simulink model "pantilt_robot"  (R2020a)
settings: Solver=VariableStepAuto  StartTime=0.0  StopTime=10.0  RelTol=1e-3
undefined symbols (not defined in the file): B, J, j, K, Kd, Ki, Kp, La, N, Ra, Ti, Tt
settings Model: Creator=nikkiepedersen  LastModifiedBy=nikkiepedersen

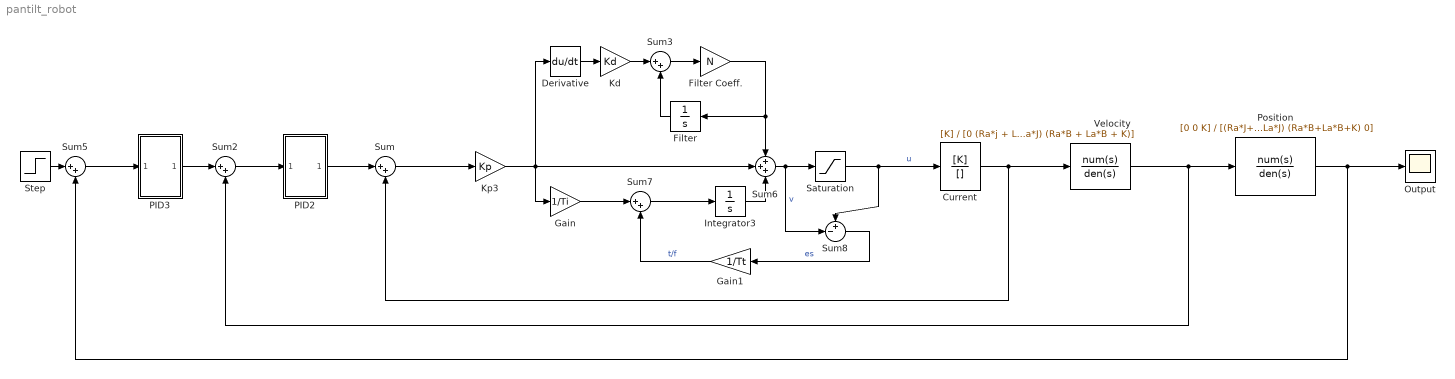
== system pantilt_robot ==
  " Kd" : Gain  Gain=Kd
  Current : TransferFcn  Numerator=[K]  Denominator=[]
  Derivative : Derivative
  Filter : Integrator
  Filter Coeff. : Gain  Gain=N
  Gain : Gain  Gain=1/Ti
  Gain1 : Gain  Gain=1/Tt
  Integrator3 : Integrator
  Kp3 : Gain  Gain=Kp
  Output : Scope
  PID2 : Subsystem
  PID3 : Subsystem
  Position : TransferFcn  Numerator=[0 0 K]  Denominator=[(Ra*J+La*J) (Ra*B+La*B+K) 0]
  Saturation : Saturate
  Step : Step  SampleTime=0
  Sum{,2..3,5,7} (5 alike) : Sum  Inputs=|++
  Sum6 : Sum  Inputs=+++
  Sum8 : Sum  Inputs=+-|
  Velocity : TransferFcn  Numerator=[K]  Denominator=[0 (Ra*j + La*J) (Ra*B + La*B + K)]
  wires:
  Sum/1 -> Kp3/1
  Current/1 -> Velocity/1, Sum/2
  Step/1 -> Sum5/1
  Velocity/1 -> Position/1, Sum2/2
  Position/1 -> Output/1, Sum5/2
  Saturation/1 -> Sum8/1, Current/1  "u"
  Sum7/1 -> Integrator3/1
  Gain/1 -> Sum7/1
  Integrator3/1 -> Sum6/3
  Sum6/1 -> Saturation/1, Sum8/2  "v"
  Sum8/1 -> Gain1/1  "es"
  Gain1/1 -> Sum7/2  "t/f"
  Sum5/1 -> PID3/1(In1)
  PID3/1(Out1) -> Sum2/1
  Sum2/1 -> PID2/1(In1)
  PID2/1(Out1) -> Sum/1
  Kp3/1 -> Derivative/1, Sum6/2, Gain/1
  " Kd"/1 -> Sum3/1
  Filter/1 -> Sum3/2
  Sum3/1 -> Filter Coeff./1
  Derivative/1 -> " Kd"/1
  Filter Coeff./1 -> Filter/1, Sum6/1

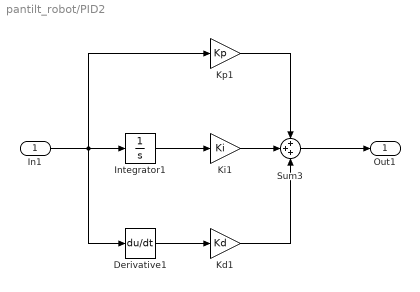
== system pantilt_robot/PID2 ==
  In1 : Inport
  Derivative1 : Derivative
  Integrator1 : Integrator
  Kd1 : Gain  Gain=Kd
  Ki1 : Gain  Gain=Ki
  Kp1 : Gain  Gain=Kp
  Sum3 : Sum  Inputs=+++
  Out1 : Outport
  wires:
  Ki1/1 -> Sum3/2
  Sum3/1 -> Out1/1
  Integrator1/1 -> Ki1/1
  Derivative1/1 -> Kd1/1
  Kp1/1 -> Sum3/1
  Kd1/1 -> Sum3/3
  In1/1 -> Derivative1/1, Kp1/1, Integrator1/1

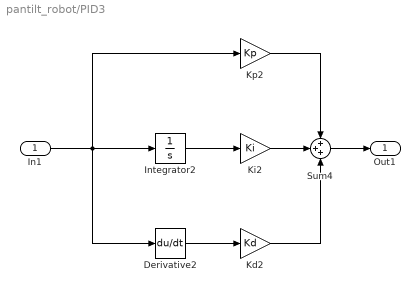
== system pantilt_robot/PID3 ==
  In1 : Inport
  Derivative2 : Derivative
  Integrator2 : Integrator
  Kd2 : Gain  Gain=Kd
  Ki2 : Gain  Gain=Ki
  Kp2 : Gain  Gain=Kp
  Sum4 : Sum  Inputs=+++
  Out1 : Outport
  wires:
  Sum4/1 -> Out1/1
  Kp2/1 -> Sum4/1
  In1/1 -> Derivative2/1, Kp2/1, Integrator2/1
  Ki2/1 -> Sum4/2
  Derivative2/1 -> Kd2/1
  Kd2/1 -> Sum4/3
  Integrator2/1 -> Ki2/1
